simulink library "rigid_body_dynamics_lib"  (R2018b)
settings: Solver=VariableStepAuto  StartTime=0.0  StopTime=10.0  RelTol=1e-3
undefined symbols (not defined in the file or in its folder): DiscIntNeverNeededParam, simParams
libraries: vrlib x1, aerolibutil x1
settings Model: Creator=taylorreynolds  LastModifiedBy=taylorreynolds

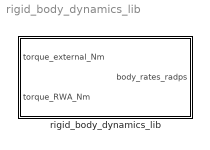
== system rigid_body_dynamics_lib ==
  rigid_body_dynamics_lib : Subsystem

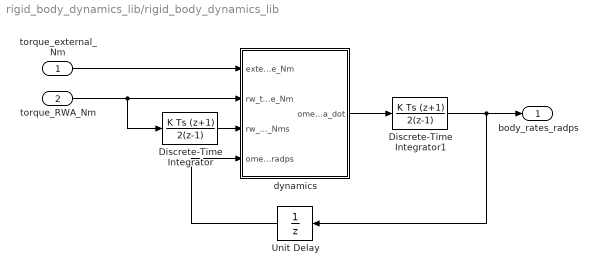
== system rigid_body_dynamics_lib/rigid_body_dynamics_lib ==
  torque_external_Nm : Inport
  torque_RWA_Nm : Inport  Port=2
  Discrete-Time Integrator : DiscreteIntegrator  IntegratorMethod=Integration: Trapezoidal  InitialCondition=simParams.initialConditions.rwa.h_body_Nms  SampleTime=-1  ICPrevOutput=DiscIntNeverNeededParam  ICPrevScaledInput=DiscIntNeverNeededParam
  Discrete-Time Integrator1 : DiscreteIntegrator  IntegratorMethod=Integration: Trapezoidal  InitialCondition=simParams.initialConditions.w_body_radps  SampleTime=-1  ICPrevOutput=DiscIntNeverNeededParam  ICPrevScaledInput=DiscIntNeverNeededParam
  Unit Delay : UnitDelay  InitialCondition=simParams.initialConditions.w_body_radps  SampleTime=-1
  dynamics : Subsystem
  body_rates_radps : Outport
  wires:
  torque_RWA_Nm/1 -> Discrete-Time Integrator/1, dynamics/2(rw_torque_Nm)
  Discrete-Time Integrator1/1 -> Unit Delay/1, body_rates_radps/1
  torque_external_Nm/1 -> dynamics/1(external_torque_Nm)
  Discrete-Time Integrator/1 -> dynamics/3(rw_momentum_Nms)
  dynamics/1(omega_dot) -> Discrete-Time Integrator1/1
  Unit Delay/1 -> dynamics/4(omega_radps)

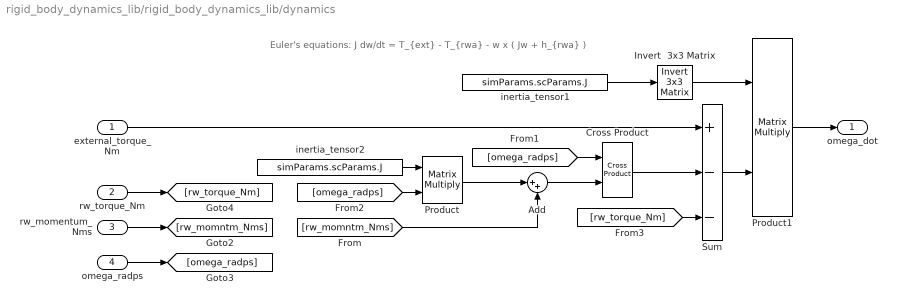
== system rigid_body_dynamics_lib/rigid_body_dynamics_lib/dynamics ==
  note: Euler's equations: J dw/dt = T_{ext} - T_{rwa} - w x ( Jw + h_{rwa} )
  external_torque_Nm : Inport
  rw_torque_Nm : Inport  Port=2
  rw_momentum_Nms : Inport  Port=3
  omega_radps : Inport  Port=4
  Add : Sum  Inputs=|++
  Cross Product : vrlib/Utilities/Cross Product
      settings: SourceProductBaseCode=VR
  Invert  3x3 Matrix : aerolibutil/Invert  3x3 Matrix
  Product : Product  Multiplication=Matrix(*)  RndMeth=Zero
  Product1 : Product  Multiplication=Matrix(*)  RndMeth=Zero
  Sum : Sum  Inputs=+--
  inertia_tensor1 : Constant  Value=simParams.scParams.J  SampleTime=simParams.sample_time_s
  inertia_tensor2 : Constant  Value=simParams.scParams.J  SampleTime=simParams.sample_time_s
  omega_dot : Outport
  wires:
  rw_torque_Nm/1 -> [rw_torque_Nm]
  Add/1 -> Cross Product/2
  Product/1 -> Add/1
  Cross Product/1 -> Sum/2
  inertia_tensor1/1 -> Invert  3x3 Matrix/1
  Invert  3x3 Matrix/1 -> Product1/1
  Product1/1 -> omega_dot/1
  Sum/1 -> Product1/2
  inertia_tensor2/1 -> Product/1
  omega_radps/1 -> [omega_radps]
  external_torque_Nm/1 -> Sum/1
  rw_momentum_Nms/1 -> [rw_momntm_Nms]
  [rw_momntm_Nms] -> Add/2
  [omega_radps] -> Cross Product/1
  [omega_radps] -> Product/2
  [rw_torque_Nm] -> Sum/3
